simulink model "SimulinkModell_for_RT_Communication"  (R2019b)
settings: Solver=ode5  StartTime=0.0  StopTime=500  RelTol=1e-3
undefined symbols (not defined in the file): Standard_Devices, UDP_Protocol
libraries: sldrtlib x6, simulink x2
settings Model: Creator=Daniel  LastModifiedBy=Daniel
settings RTWCC: Description=Simulink Desktop Real-Time  SystemTargetFile=sldrt.tlc  TemplateMakefile=sldrt.tmf  RTWCompilerOptimization=on
settings CodeAppCC: MaxIdLength=95
settings SimulinkDesktopRealTimeCC: TargetPreCompLibLocation=D:\MatLab\toolbox\sldrt\lib\win64  PreserveStateflowLocalDataDimensions=off

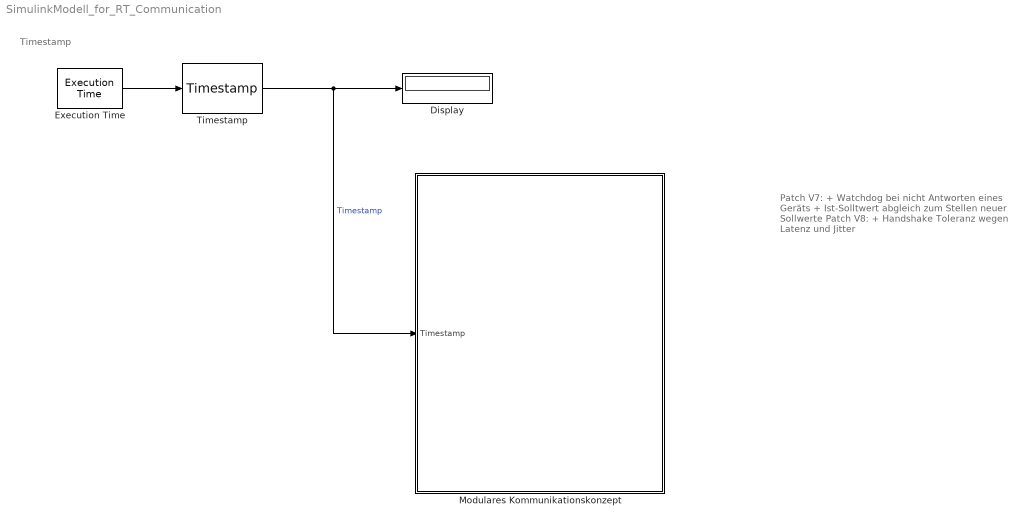
== system SimulinkModell_for_RT_Communication ==
  note: Patch V7:
      | + Watchdog bei nicht Antworten eines Geräts
      | + Ist-Solltwert abgleich zum Stellen neuer Sollwerte
      |
      | Patch V8:
      | + Handshake Toleranz wegen Latenz und Jitter
  note: Timestamp
  Display : Display
  Execution Time : sldrtlib/Target Profiling/Execution Time  ShowTaskTimes=off
      settings: SourceProductName=Simulink Desktop Real-Time  SourceProductBaseCode=WT
  Modulares Kommunikationskonzept : Subsystem
  Timestamp : sldrtlib/Target Profiling/Timestamp
      settings: SourceProductName=Simulink Desktop Real-Time  SourceProductBaseCode=WT
  wires:
  Timestamp/1 -> Modulares Kommunikationskonzept/1(Timestamp), Display/1  "Timestamp"
  Execution Time/1 -> Timestamp/1

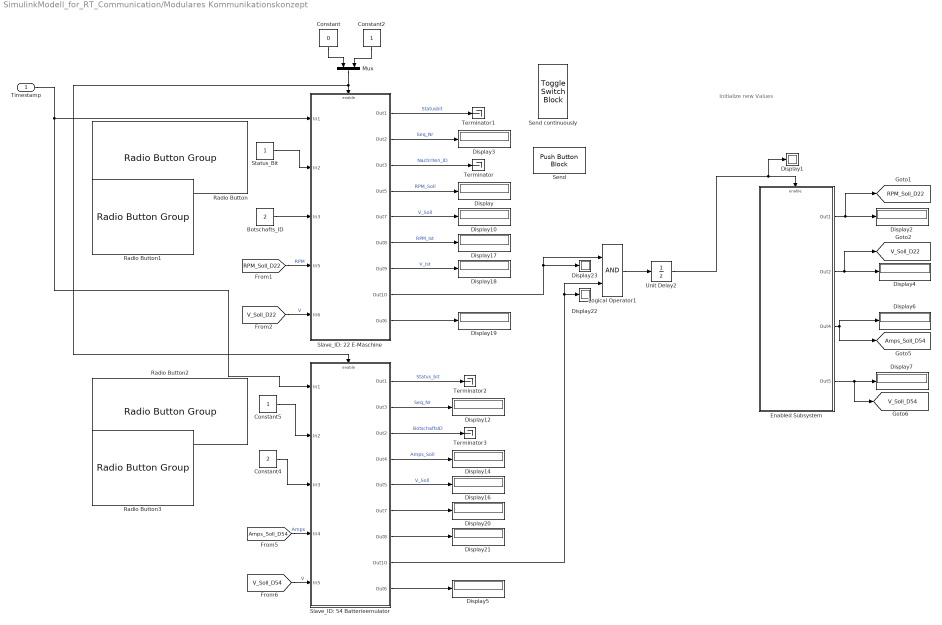
== system SimulinkModell_for_RT_Communication/Modulares Kommunikationskonzept ==
  note: Initialize new Values
  Timestamp : Inport
  Botschafts_ID : Constant  Value=2
  Constant : Constant  Value=0
  Constant2 : Constant
  Constant4 : Constant  Value=2
  Constant5 : Constant
  Display{,1..7,10,12,14,16..23} (19 alike) : Display
  Enabled Subsystem : Subsystem  TreatAsAtomicUnit=on
  Logical Operator1 : Logic  AllPortsSameDT=off  OutDataTypeStr=boolean
  Mux : Mux  Inputs=2
  Radio Button : RadioButtonGroup  LabelPosition=Hide  SelectedLabel=Response_Simulation_D22  ButtonGroupName=Status_Bit
      settings: Values={{'NoResponse_Simulation_D22', 'Response_Simulation_D22'}, [0 1]}
  Radio Button1 : RadioButtonGroup  LabelPosition=Hide  SelectedLabel=Datenabfrage_ID  ButtonGroupName=Botschafts_IDs
      settings: Values={{'Sollwert_ID', 'Datenabfrage_ID', 'Config_ID'}, [1 2 3]}
  Radio Button2 : RadioButtonGroup  LabelPosition=Hide  SelectedLabel=Response_Simulation_D54  ButtonGroupName=Status_Bit
      settings: Values={{'NoResponse_Simulation_D54', 'Response_Simulation_D54'}, [0 1]}
  Radio Button3 : RadioButtonGroup  LabelPosition=Hide  SelectedLabel=Datenabfrage_ID  ButtonGroupName=Botschafts_IDs
      settings: Values={{'Sollwert_ID', 'Datenabfrage_ID', 'Config_ID'}, [1 2 3]}
  Send : PushButtonBlock  ButtonText=Senden
  Send continuously : ToggleSwitchBlock  LabelPosition=Hide
      settings: Values={{'Off', 'On'}, [0 1]}
  Slave_ID: 22 E-Maschine : Subsystem  TreatAsAtomicUnit=on
  Slave_ID: 54 Batterieemulator : Subsystem  TreatAsAtomicUnit=on
  Status_Bit : Constant
  Terminator{,1..3} (4 alike) : Terminator
  Unit Delay2 : UnitDelay  InitialCondition=1  InputProcessing=Columns as channels (frame based)  SampleTime=-1  HasFrameUpgradeWarning=on
  tag scope: Amps_Soll_D54=global, RPM_Soll_D22=global, V_Soll_D22=global, V_Soll_D54=global
  wires:
  Timestamp/1 -> Slave_ID: 22 E-Maschine/1(In1), Slave_ID: 54 Batterieemulator/1(In1)
  Enabled Subsystem/4(Out5) -> Display7/1, [V_Soll_D54]
  Enabled Subsystem/1(Out1) -> [RPM_Soll_D22], Display2/1
  Enabled Subsystem/3(Out4) -> Display6/1, [Amps_Soll_D54]
  Slave_ID: 54 Batterieemulator/1(Out1) -> Terminator2/1  "Status_bit"
  Slave_ID: 22 E-Maschine/1(Out1) -> Terminator1/1  "Statusbit"
  Enabled Subsystem/2(Out2) -> Display4/1, [V_Soll_D22]
  [V_Soll_D54] -> Slave_ID: 54 Batterieemulator/5(In5)  "V"
  Constant/1 -> Mux/1
  [RPM_Soll_D22] -> Slave_ID: 22 E-Maschine/4(In5)  "RPM"
  [V_Soll_D22] -> Slave_ID: 22 E-Maschine/5(In6)  "V"
  Slave_ID: 22 E-Maschine/2(Out2) -> Display3/1  "Seq_Nr"
  Constant5/1 -> Slave_ID: 54 Batterieemulator/2(In2)
  Slave_ID: 22 E-Maschine/3(Out3) -> Terminator/1  "Nachriten_ID"
  Status_Bit/1 -> Slave_ID: 22 E-Maschine/2(In2)
  [Amps_Soll_D54] -> Slave_ID: 54 Batterieemulator/4(In4)  "Amps"
  Slave_ID: 54 Batterieemulator/2(Out3) -> Display12/1  "Seq_Nr"
  Slave_ID: 54 Batterieemulator/4(Out4) -> Display14/1  "Amps_Soll"
  Slave_ID: 54 Batterieemulator/3(Out2) -> Terminator3/1  "BotschaftsID"
  Logical Operator1/1 -> Unit Delay2/1
  Slave_ID: 22 E-Maschine/4(Out5) -> Display/1  "RPM_Soll"
  Slave_ID: 54 Batterieemulator/5(Out5) -> Display16/1  "V_Soll"
  Slave_ID: 22 E-Maschine/9(Out6) -> Display19/1
  Constant2/1 -> Mux/2
  Mux/1 -> Slave_ID: 54 Batterieemulator/Enable, Slave_ID: 22 E-Maschine/Enable
  Botschafts_ID/1 -> Slave_ID: 22 E-Maschine/3("In3 ")
  Slave_ID: 22 E-Maschine/5(Out7) -> Display10/1  "V_Soll"
  Slave_ID: 22 E-Maschine/6(Out8) -> Display17/1  "RPM_Ist"
  Slave_ID: 22 E-Maschine/7(Out9) -> Display18/1  "V_Ist"
  Constant4/1 -> Slave_ID: 54 Batterieemulator/3(In3)
  Slave_ID: 54 Batterieemulator/6(Out7) -> Display20/1
  Slave_ID: 54 Batterieemulator/7(Out8) -> Display21/1
  Slave_ID: 54 Batterieemulator/8(Out10) -> Logical Operator1/2, Display22/1
  Slave_ID: 22 E-Maschine/8(Out10) -> Logical Operator1/1, Display23/1
  Slave_ID: 54 Batterieemulator/9(Out6) -> Display5/1
  Unit Delay2/1 -> Display1/1, Enabled Subsystem/Enable

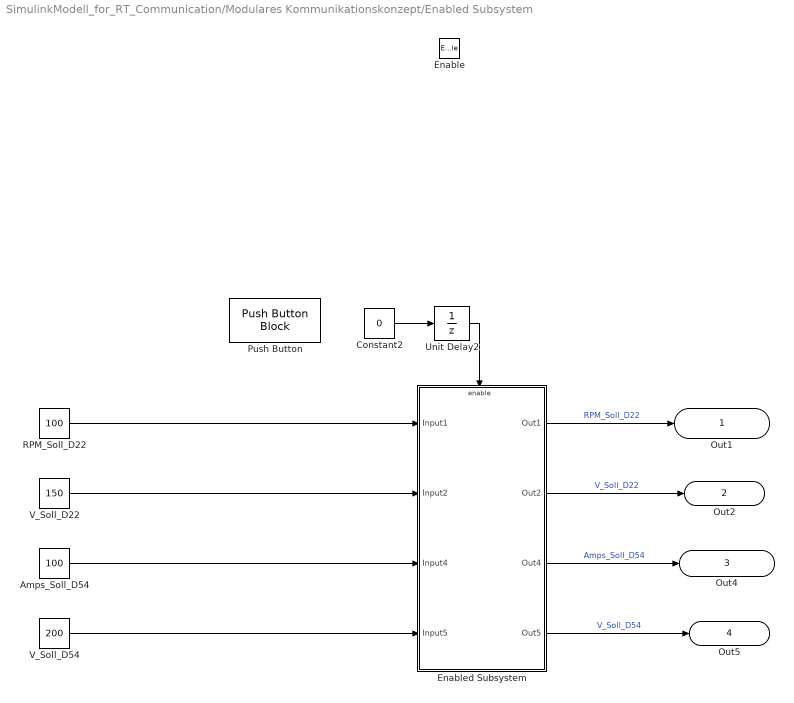
== system SimulinkModell_for_RT_Communication/Modulares Kommunikationskonzept/Enabled Subsystem ==
  Enable : EnablePort
  Amps_Soll_D54 : Constant  Value=100  SampleTime=0.1
  Constant2 : Constant  Value=0
  Enabled Subsystem : Subsystem  TreatAsAtomicUnit=on
  Push Button : PushButtonBlock  ButtonText=Initialisieren
  RPM_Soll_D22 : Constant  Value=100  SampleTime=0.1
  Unit Delay2 : UnitDelay  InitialCondition=1  InputProcessing=Columns as channels (frame based)  SampleTime=-1  HasFrameUpgradeWarning=on
  V_Soll_D22 : Constant  Value=150  SampleTime=0.1
  V_Soll_D54 : Constant  Value=200  SampleTime=0.1
  Out1 : Outport
  Out2 : Outport  Port=2
  Out4 : Outport  Port=3
  Out5 : Outport  Port=4
  wires:
  V_Soll_D22/1 -> Enabled Subsystem/2(Input2)
  RPM_Soll_D22/1 -> Enabled Subsystem/1(Input1)
  Enabled Subsystem/2("Out2 ") -> Out2/1  "V_Soll_D22"
  Enabled Subsystem/1(Out1) -> Out1/1  "RPM_Soll_D22"
  Amps_Soll_D54/1 -> Enabled Subsystem/3(Input4)
  V_Soll_D54/1 -> Enabled Subsystem/4(Input5)
  Enabled Subsystem/3(Out4) -> Out4/1  "Amps_Soll_D54"
  Enabled Subsystem/4(Out5) -> Out5/1  "V_Soll_D54"
  Constant2/1 -> Unit Delay2/1
  Unit Delay2/1 -> Enabled Subsystem/Enable

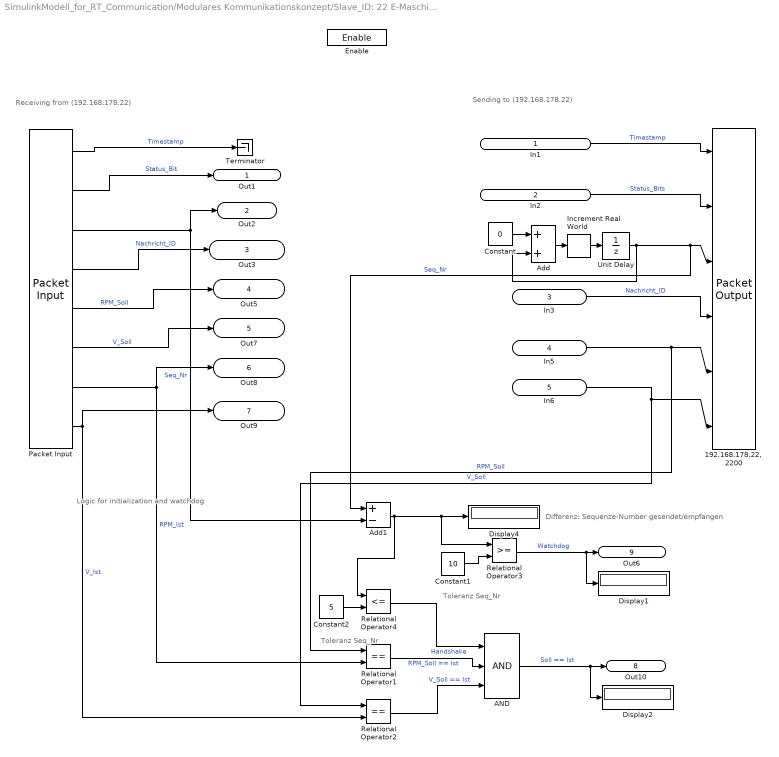
== system SimulinkModell_for_RT_Communication/Modulares Kommunikationskonzept/Slave_ID: 22 E-Maschine ==
  note: Differenz: Sequenze-Number gesendet/empfangen
  note: Toleranz Seq_Nr
  note: Logic for initialization and watchdog
  note: Sending to (192.168.178.22)
  note: Receiving from (192.168.178.22)
  note: Toleranz Seq_Nr
  In1 : Inport
  In2 : Inport  Port=2
  "In3 " : Inport  Port=3
  In5 : Inport  Port=4
  In6 : Inport  Port=5
  Enable : EnablePort
  "192.168.178.22, 2200" : sldrtlib/Packet Output  SampleTime=0.5  MaxMissedTicks=10  ShowMissedTicks=off  YieldWhenWaiting=off  DrvName=Standard_Devices/UDP_Protocol  DrvAddress=22  DrvOptions=[0 2200 49 57 50 46 49 54 56 46 49 55 56 46 50 50 0 0 0 0 0 0 0 0 0 0 0 0 0 0 0 0 0 0 0 0 0 0 0 0 0 0 0 0 0 0 0 0 0 0 0 0 0 0 0 0 0 0 0 0 0 0 0 0 0 0 0 0 0 0 0 0 0 0 0 0 0 0 0 0 0 0 0 0 0 0 0 0 0 0 0 0 0 0 0 0 0 0 0 0 0 0 0 0 0 0 0 0 0 0 0 0 0 0 0 0 0 0 0 0 0 0 0 0 0 0 0 0 0 0 0 0 0 0 0 0 0 0 0 0 0 0 0 0 0 0 0 0 0 0 0 0 0 0 0 0 0 0 0 0 0 0 0 0 0 0 0 0 0 0 0 0 0 0 0 0 0 0 0 0 0 0 0 0 0 0 0 0 0 0 0 0 0 0 0 0 0 0 0 0 0 0 0 0 0 0 0 0 0 0 0 0 0 0 0 0 0 0 0 0 0 0 0 0 0 0 0 0 0 0 0 0 0 0 0 0 0 0 0 0 0 0 0 0 0 0 0 0 0 0 0 0 0 0 0 0]  PacketSize=(6*4)  DataTypes={'1*single','1*single','1*single','1*single','1*single','1*single'}  ShowReady=off  ShowError=off  PacketID=1  ByteOrder=1  InitialValue=[]  FinalValue=[]
      settings: AttributesFormatString=UDP Protocol [22]  SourceProductName=Simulink Desktop Real-Time
  AND : Logic  Inputs=3  AllPortsSameDT=off  OutDataTypeStr=boolean
  Add : Sum  OutDataTypeStr=single
  Add1 : Sum  Inputs=+-
  Constant : Constant  Value=0  OutDataTypeStr=single  SampleTime=0.5
  Constant1 : Constant  Value=10
  Constant2 : Constant  Value=5
  Display1 : Display
  Display2 : Display
  Display4 : Display
  Increment Real World : simulink/Additional Math & Discrete/Additional Math: Increment - Decrement/Increment Real World
      settings: SourceProductName=Simulink  SourceProductBaseCode=SL
  Packet Input : sldrtlib/Packet Input  SampleTime=0.0001  MaxMissedTicks=10  ShowMissedTicks=off  YieldWhenWaiting=off  DrvName=Standard_Devices/UDP_Protocol  DrvAddress=22  DrvOptions=[0 2200 49 57 50 46 49 54 56 46 49 55 56 46 50 50 0 0 0 0 0 0 0 0 0 0 0 0 0 0 0 0 0 0 0 0 0 0 0 0 0 0 0 0 0 0 0 0 0 0 0 0 0 0 0 0 0 0 0 0 0 0 0 0 0 0 0 0 0 0 0 0 0 0 0 0 0 0 0 0 0 0 0 0 0 0 0 0 0 0 0 0 0 0 0 0 0 0 0 0 0 0 0 0 0 0 0 0 0 0 0 0 0 0 0 0 0 0 0 0 0 0 0 0 0 0 0 0 0 0 0 0 0 0 0 0 0 0 0 0 0 0 0 0 0 0 0 0 0 0 0 0 0 0 0 0 0 0 0 0 0 0 0 0 0 0 0 0 0 0 0 0 0 0 0 0 0 0 0 0 0 0 0 0 0 0 0 0 0 0 0 0 0 0 0 0 0 0 0 0 0 0 0 0 0 0 0 0 0 0 0 0 0 0 0 0 0 0 0 0 0 0 0 0 0 0 0 0 0 0 0 0 0 0 0 0 0 0 0 0 0 0 0 0 0 0 0 0 0 0 0 0 0 0 0 0]  PacketSize=(8*4)  DataTypes={'1*single','1*single','1*single','1*single','1*single','1*single','1*single','1*single'}  ShowReady=off  ShowError=off  PacketID=1  ByteOrder=1  ShowTimestamp=off
      settings: AttributesFormatString=UDP Protocol [22]  SourceProductName=Simulink Desktop Real-Time
  Relational Operator1 : RelationalOperator  Operator===  OutDataTypeStr=boolean  RndMeth=Simplest
  Relational Operator2 : RelationalOperator  Operator===  OutDataTypeStr=boolean  RndMeth=Simplest
  Relational Operator3 : RelationalOperator  OutDataTypeStr=boolean  RndMeth=Simplest
  Relational Operator4 : RelationalOperator  Operator=<=  OutDataTypeStr=boolean  RndMeth=Simplest
  Terminator : Terminator
  Unit Delay : UnitDelay  InitialCondition=1  SampleTime=-1  HasFrameUpgradeWarning=on
  Out1 : Outport
  Out2 : Outport  Port=2
  Out3 : Outport  Port=3
  Out5 : Outport  Port=4
  Out7 : Outport  Port=5
  Out8 : Outport  Port=6
  Out9 : Outport  Port=7
  Out10 : Outport  Port=8
  Out6 : Outport  Port=9
  wires:
  In1/1 -> "192.168.178.22, 2200"/1  "Timestamp"
  In2/1 -> "192.168.178.22, 2200"/2  "Status_Bits"
  In5/1 -> "192.168.178.22, 2200"/5, Relational Operator1/1  "RPM_Soll"
  "In3 "/1 -> "192.168.178.22, 2200"/4  "Nachricht_ID"
  Packet Input/3 -> Out2/1, Add1/2  "Seq_Nr"
  Packet Input/1 -> Terminator/1  "Timestamp"
  Packet Input/2 -> Out1/1  "Status_Bit"
  Packet Input/4 -> Out3/1  "Nachricht_ID"
  In6/1 -> "192.168.178.22, 2200"/6, Relational Operator2/1  "V_Soll"
  Packet Input/7 -> Out8/1, Relational Operator1/2  "RPM_Ist"
  Packet Input/8 -> Out9/1, Relational Operator2/2  "V_Ist"
  Packet Input/5 -> Out5/1  "RPM_Soll"
  Packet Input/6 -> Out7/1  "V_Soll"
  Add/1 -> Increment Real World/1
  Constant/1 -> Add/1
  Unit Delay/1 -> Add1/1, "192.168.178.22, 2200"/3, Add/2  "Seq_Nr"
  Increment Real World/1 -> Unit Delay/1
  Relational Operator4/1 -> AND/1  "Handshake"
  Relational Operator1/1 -> AND/2  "RPM_Soll == Ist"
  Relational Operator2/1 -> AND/3  "V_Soll == Ist"
  AND/1 -> Display2/1, Out10/1  "Soll == Ist"
  Constant1/1 -> Relational Operator3/2
  Add1/1 -> Relational Operator4/1, Relational Operator3/1, Display4/1
  Relational Operator3/1 -> Display1/1, Out6/1  "Watchdog"
  Constant2/1 -> Relational Operator4/2

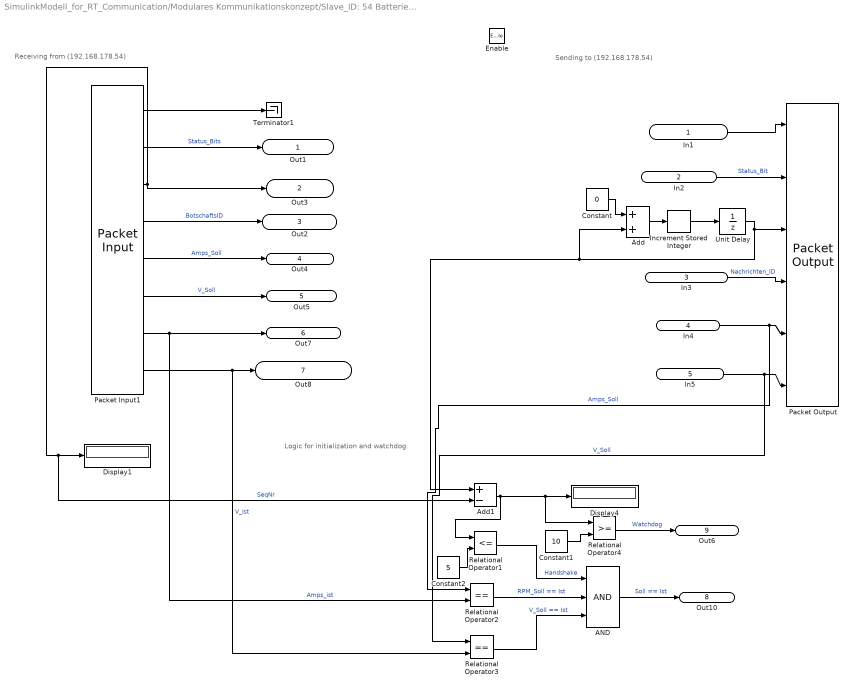
== system SimulinkModell_for_RT_Communication/Modulares Kommunikationskonzept/Slave_ID: 54 Batterieemulator ==
  note: Logic for initialization and watchdog
  note: Sending to (192.168.178.54)
  note: Receiving from (192.168.178.54)
  In1 : Inport
  In2 : Inport  Port=2
  In3 : Inport  Port=3
  In4 : Inport  Port=4
  In5 : Inport  Port=5
  Enable : EnablePort
  AND : Logic  Inputs=3  AllPortsSameDT=off  OutDataTypeStr=boolean
  Add : Sum
  Add1 : Sum  Inputs=+-
  Constant : Constant  Value=0  SampleTime=0.5
  Constant1 : Constant  Value=10
  Constant2 : Constant  Value=5
  Display1 : Display
  Display4 : Display
  Increment Stored Integer : simulink/Additional Math & Discrete/Additional Math: Increment - Decrement/Increment Stored Integer
      settings: SourceProductName=Simulink
  Packet Input1 : sldrtlib/Packet Input  SampleTime=0.0001  MaxMissedTicks=10  ShowMissedTicks=off  YieldWhenWaiting=off  DrvName=Standard_Devices/UDP_Protocol  DrvAddress=54  DrvOptions=[0 5400 49 57 50 46 49 54 56 46 49 55 56 46 53 52 0 0 0 0 0 0 0 0 0 0 0 0 0 0 0 0 0 0 0 0 0 0 0 0 0 0 0 0 0 0 0 0 0 0 0 0 0 0 0 0 0 0 0 0 0 0 0 0 0 0 0 0 0 0 0 0 0 0 0 0 0 0 0 0 0 0 0 0 0 0 0 0 0 0 0 0 0 0 0 0 0 0 0 0 0 0 0 0 0 0 0 0 0 0 0 0 0 0 0 0 0 0 0 0 0 0 0 0 0 0 0 0 0 0 0 0 0 0 0 0 0 0 0 0 0 0 0 0 0 0 0 0 0 0 0 0 0 0 0 0 0 0 0 0 0 0 0 0 0 0 0 0 0 0 0 0 0 0 0 0 0 0 0 0 0 0 0 0 0 0 0 0 0 0 0 0 0 0 0 0 0 0 0 0 0 0 0 0 0 0 0 0 0 0 0 0 0 0 0 0 0 0 0 0 0 0 0 0 0 0 0 0 0 0 0 0 0 0 0 0 0 0 0 0 0 0 0 0 0 0 0 0 0 0 0 0 0 0 0 0]  PacketSize=(8*4)  DataTypes={'1*single','1*single','1*single','1*single','1*single','1*single','1*single','1*single'}  ShowReady=off  ShowError=off  PacketID=1  ByteOrder=1  ShowTimestamp=off
      settings: AttributesFormatString=UDP Protocol [54]  SourceProductName=Simulink Desktop Real-Time
  Packet Output : sldrtlib/Packet Output  SampleTime=0.5  MaxMissedTicks=10  ShowMissedTicks=off  YieldWhenWaiting=off  DrvName=Standard_Devices/UDP_Protocol  DrvAddress=54  DrvOptions=[0 5400 49 57 50 46 49 54 56 46 49 55 56 46 53 52 0 0 0 0 0 0 0 0 0 0 0 0 0 0 0 0 0 0 0 0 0 0 0 0 0 0 0 0 0 0 0 0 0 0 0 0 0 0 0 0 0 0 0 0 0 0 0 0 0 0 0 0 0 0 0 0 0 0 0 0 0 0 0 0 0 0 0 0 0 0 0 0 0 0 0 0 0 0 0 0 0 0 0 0 0 0 0 0 0 0 0 0 0 0 0 0 0 0 0 0 0 0 0 0 0 0 0 0 0 0 0 0 0 0 0 0 0 0 0 0 0 0 0 0 0 0 0 0 0 0 0 0 0 0 0 0 0 0 0 0 0 0 0 0 0 0 0 0 0 0 0 0 0 0 0 0 0 0 0 0 0 0 0 0 0 0 0 0 0 0 0 0 0 0 0 0 0 0 0 0 0 0 0 0 0 0 0 0 0 0 0 0 0 0 0 0 0 0 0 0 0 0 0 0 0 0 0 0 0 0 0 0 0 0 0 0 0 0 0 0 0 0 0 0 0 0 0 0 0 0 0 0 0 0 0 0 0 0 0 0]  PacketSize=(6*4)  DataTypes={'1*single','1*single','1*single','1*single','1*single','1*single'}  ShowReady=off  ShowError=off  PacketID=1  ByteOrder=1  InitialValue=[]  FinalValue=[]
      settings: AttributesFormatString=UDP Protocol [54]  SourceProductName=Simulink Desktop Real-Time
  Relational Operator1 : RelationalOperator  Operator=<=  OutDataTypeStr=boolean  RndMeth=Simplest
  Relational Operator2 : RelationalOperator  Operator===  OutDataTypeStr=boolean  RndMeth=Simplest
  Relational Operator3 : RelationalOperator  Operator===  OutDataTypeStr=boolean  RndMeth=Simplest
  Relational Operator4 : RelationalOperator  OutDataTypeStr=boolean  RndMeth=Simplest
  Terminator1 : Terminator
  Unit Delay : UnitDelay  InitialCondition=1  SampleTime=-1  HasFrameUpgradeWarning=on
  Out1 : Outport
  Out3 : Outport  Port=2
  Out2 : Outport  Port=3
  Out4 : Outport  Port=4
  Out5 : Outport  Port=5
  Out7 : Outport  Port=6
  Out8 : Outport  Port=7
  Out10 : Outport  Port=8
  Out6 : Outport  Port=9
  wires:
  In1/1 -> Packet Output/1
  In2/1 -> Packet Output/2  "Status_Bit"
  In3/1 -> Packet Output/4  "Nachrichten_ID"
  In4/1 -> Relational Operator2/1, Packet Output/5  "Amps_Soll"
  In5/1 -> Relational Operator3/1, Packet Output/6  "V_Soll"
  Packet Input1/5 -> Out4/1  "Amps_Soll"
  Packet Input1/1 -> Terminator1/1
  Packet Input1/3 -> Out3/1, Add1/2, Display1/1  "SeqNr"
  Packet Input1/4 -> Out2/1  "BotschaftsID"
  Packet Input1/2 -> Out1/1  "Status_Bits"
  Increment Stored Integer/1 -> Unit Delay/1
  Constant/1 -> Add/1
  Unit Delay/1 -> Add1/1, Add/2, Packet Output/3
  Relational Operator1/1 -> AND/1  "Handshake"
  Packet Input1/6 -> Out5/1  "V_Soll"
  Packet Input1/7 -> Relational Operator2/2, Out7/1  "Amps_ist"
  Packet Input1/8 -> Relational Operator3/2, Out8/1  "V_Ist"
  Relational Operator2/1 -> AND/2  "RPM_Soll == Ist"
  Relational Operator3/1 -> AND/3  "V_Soll == Ist"
  AND/1 -> Out10/1  "Soll == Ist"
  Add/1 -> Increment Stored Integer/1
  Add1/1 -> Relational Operator1/1, Relational Operator4/1, Display4/1
  Relational Operator4/1 -> Out6/1  "Watchdog"
  Constant1/1 -> Relational Operator4/2
  Constant2/1 -> Relational Operator1/2

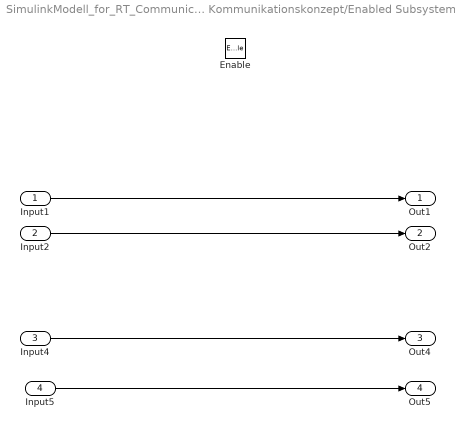
== system SimulinkModell_for_RT_Communication/Modulares Kommunikationskonzept/Enabled Subsystem/Enabled Subsystem ==
  Input1 : Inport
  Input2 : Inport  Port=2
  Input4 : Inport  Port=3
  Input5 : Inport  Port=4
  Enable : EnablePort
  Out1 : Outport
  "Out2 " : Outport  Port=2
  Out4 : Outport  Port=3
  Out5 : Outport  Port=4
  wires:
  Input1/1 -> Out1/1
  Input2/1 -> "Out2 "/1
  Input4/1 -> Out4/1
  Input5/1 -> Out5/1
